simulink subsystem "EEG_Ratio_Model"  (R2020a)
settings: Solver=VariableStepAuto  StartTime=0.0  StopTime=10.0  RelTol=1e-3
settings Model: Creator=LAB-OREN3  LastModifiedBy=LAB-OREN3

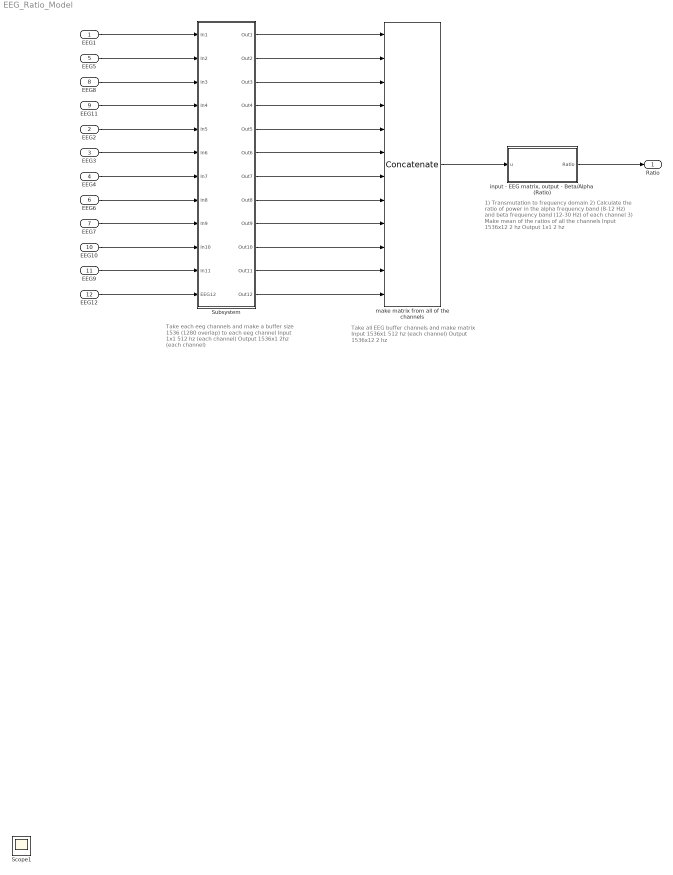
== system EEG_Ratio_Model ==
  note: Take each eeg channels and make a buffer size 1536 (1280 overlap) to each eeg channel
      |
      | Input 1x1 512 hz (each channel)
      | Output 1536x1 2hz (each channel)
  note: Take all EEG buffer channels and make matrix
      |
      | Input 1536x1 512 hz (each channel)
      | Output 1536x12 2 hz
  note: 1) Transmutation to frequency domain
      |
      | 2) Calculate the ratio of power in the alpha frequency band (8-12 Hz) and beta frequency band (12-30 Hz) of each channel
      |
      | 3) Make mean of the ratios of all the channels
      |
      | Input 1536x12 2 hz
      | Output 1x1 2 hz
  EEG1 : Inport
  EEG2 : Inport  Port=2
  EEG3 : Inport  Port=3
  EEG4 : Inport  Port=4
  EEG5 : Inport  Port=5
  EEG6 : Inport  Port=6
  EEG7 : Inport  Port=7
  EEG8 : Inport  Port=8
  EEG11 : Inport  Port=9
  EEG10 : Inport  Port=10
  EEG9 : Inport  Port=11
  EEG12 : Inport  Port=12
  Scope1 : Scope
  Subsystem : Subsystem
  "input - EEG matrix, output - Beta/Alpha (Ratio)" : MATLAB Function  TreatAsAtomicUnit=on
  make matrix from all of the channels : Concatenate  NumInputs=12  Mode=Multidimensional array  ConcatenateDimension=2
  Ratio : Outport
  wires:
  make matrix from all of the channels/1 -> "input - EEG matrix, output - Beta/Alpha (Ratio)"/1(u)
  EEG1/1 -> Subsystem/1(In1)
  EEG5/1 -> Subsystem/2(In2)
  EEG8/1 -> Subsystem/3(In3)
  EEG11/1 -> Subsystem/4(In4)
  EEG2/1 -> Subsystem/5(In5)
  EEG3/1 -> Subsystem/6(In6)
  EEG4/1 -> Subsystem/7(In7)
  EEG6/1 -> Subsystem/8(In8)
  EEG7/1 -> Subsystem/9(In9)
  EEG10/1 -> Subsystem/10(In10)
  EEG9/1 -> Subsystem/11(In11)
  Subsystem/1(Out1) -> make matrix from all of the channels/1
  Subsystem/2(Out2) -> make matrix from all of the channels/2
  Subsystem/3(Out3) -> make matrix from all of the channels/3
  Subsystem/4(Out4) -> make matrix from all of the channels/4
  Subsystem/5(Out5) -> make matrix from all of the channels/5
  Subsystem/6(Out6) -> make matrix from all of the channels/6
  Subsystem/7(Out7) -> make matrix from all of the channels/7
  Subsystem/8(Out8) -> make matrix from all of the channels/8
  Subsystem/9(Out9) -> make matrix from all of the channels/9
  Subsystem/10(Out10) -> make matrix from all of the channels/10
  Subsystem/11(Out11) -> make matrix from all of the channels/11
  "input - EEG matrix, output - Beta/Alpha (Ratio)"/1(Ratio) -> Ratio/1
  EEG12/1 -> Subsystem/12(EEG12)
  Subsystem/12(Out12) -> make matrix from all of the channels/12

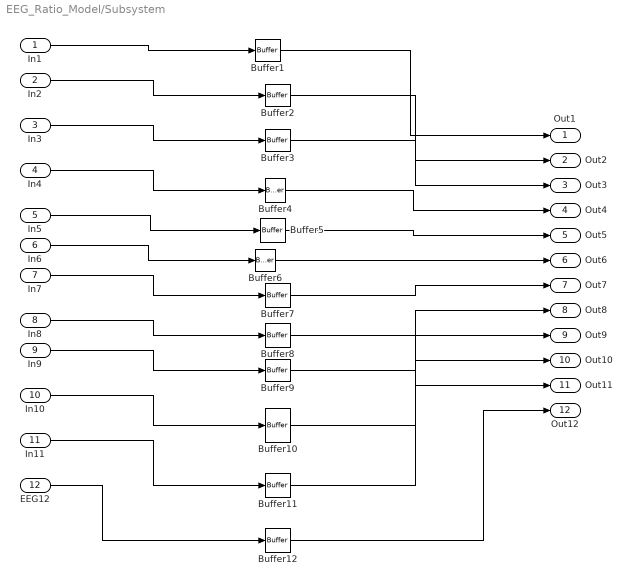
== system EEG_Ratio_Model/Subsystem ==
  In1 : Inport
  In2 : Inport  Port=2
  In3 : Inport  Port=3
  In4 : Inport  Port=4
  In5 : Inport  Port=5
  In6 : Inport  Port=6
  In7 : Inport  Port=7
  In8 : Inport  Port=8
  In9 : Inport  Port=9
  In10 : Inport  Port=10
  In11 : Inport  Port=11
  EEG12 : Inport  Port=12
  Buffer{1..12} (12 alike) : Buffer  N=1536  V=1280  OutputFrames=off
  Out1 : Outport
  Out2 : Outport  Port=2
  Out3 : Outport  Port=3
  Out4 : Outport  Port=4
  Out5 : Outport  Port=5
  Out6 : Outport  Port=6
  Out7 : Outport  Port=7
  Out8 : Outport  Port=8
  Out9 : Outport  Port=9
  Out10 : Outport  Port=10
  Out11 : Outport  Port=11
  Out12 : Outport  Port=12
  wires:
  Buffer12/1 -> Out12/1
  EEG12/1 -> Buffer12/1
  In11/1 -> Buffer11/1
  In5/1 -> Buffer5/1
  In7/1 -> Buffer7/1
  Buffer2/1 -> Out2/1
  In3/1 -> Buffer3/1
  In2/1 -> Buffer2/1
  In8/1 -> Buffer8/1
  In4/1 -> Buffer4/1
  In10/1 -> Buffer10/1
  Buffer5/1 -> Out5/1
  Buffer10/1 -> Out10/1
  Buffer11/1 -> Out11/1
  In6/1 -> Buffer6/1
  Buffer1/1 -> Out1/1
  Buffer4/1 -> Out4/1
  Buffer8/1 -> Out8/1
  Buffer7/1 -> Out7/1
  In1/1 -> Buffer1/1
  Buffer3/1 -> Out3/1
  Buffer6/1 -> Out6/1
  In9/1 -> Buffer9/1
  Buffer9/1 -> Out9/1

== matlab function EEG_Ratio_Model/input - EEG matrix, output - Beta//Alpha (Ratio) ==
  data: u input; Ratio output
function Ratio = EEG_Stress_Ratio(u)

Ratio= eeg_stress_ratio(u);


end
